simulink model "gyroControlRecpPhase"  (R2021b)
settings: Solver=FixedStepAuto  StartTime=0.0  StopTime=10.0  FixedStep=1e-4  RelTol=1e-3
values from neighbouring files (symbols this model uses):
  tau = L/v    (= 4.58549932353e-06)    [gyroControlDemod.m]    (also in gyroControlPhaseUnmod.m; gyroDigControlDemod.m; gyroModulationsExample.m; gyroSakajiri2008.m)
settings Model: Creator=Stinky  LastModifiedBy=Stinky

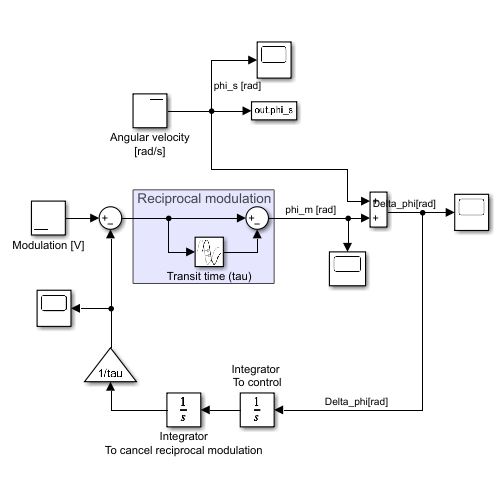
[thumbnail: Simulink's stored preview of the top-level diagram]
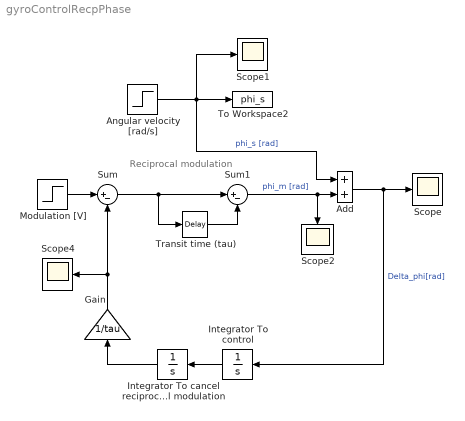
== system gyroControlRecpPhase ==
  note: Reciprocal modulation
  Add : Sum
  Angular velocity [rad/s] : Step  SampleTime=0
  Gain : Gain  Gain=1/tau
  Integrator To cancel reciprocal modulation : Integrator
  Integrator To control : Integrator
  Modulation [V] : Step  Time=0  After=0  SampleTime=0
  Scope{,1..2,4} (4 alike) : Scope
  Sum : Sum  Inputs=|+-
  Sum1 : Sum  Inputs=|+-
  To Workspace2 : ToWorkspace  VariableName=phi_s  SaveFormat=Timeseries  SampleTime=-1
  Transit time (tau) : TransportDelay  DelayTime=tau
  wires:
  Angular velocity [rad/s]/1 -> Scope1/1, To Workspace2/1, Add/1  "phi_s [rad]"
  Modulation [V]/1 -> Sum/1
  Add/1 -> Integrator To control/1, Scope/1  "Delta_phi[rad]"
  Integrator To control/1 -> Integrator To cancel reciprocal modulation/1
  Sum1/1 -> Scope2/1, Add/2  "phi_m [rad]"
  Integrator To cancel reciprocal modulation/1 -> Gain/1
  Transit time (tau)/1 -> Sum1/2
  Sum/1 -> Sum1/1, Transit time (tau)/1
  Gain/1 -> Sum/2, Scope4/1
